simulink model "Signalmodulation"  (R2024b)
settings: Solver=VariableStepAuto  StartTime=0.0  StopTime=10.0  RelTol=1e-3
libraries: commchan3 x1, simulink x1, dspfdesign x1
settings Model: Creator=pc  LastModifiedBy=pc
settings DebuggingCC: UnconnectedInputMsg=warning  UnconnectedOutputMsg=warning  UnconnectedLineMsg=warning
settings ModelReferenceCC: EnableRefExpFcnMdlSchedulingChecks=on
settings RTWCC: GPUComputeCapability=3.5  DLArmComputeVersion=19.05

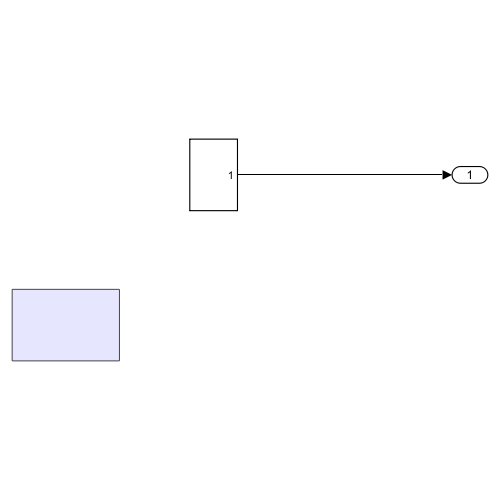
[thumbnail: Simulink's stored preview of the top-level diagram]
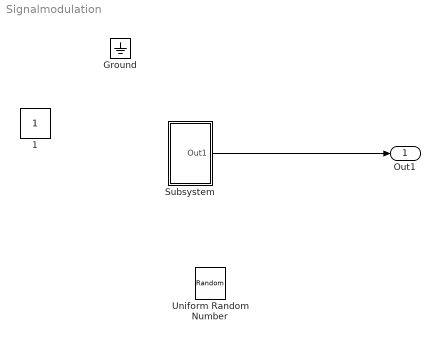
== system Signalmodulation ==
  Subsystem : Subsystem
  Out1 : Outport
  "1 " : Constant  IOType=siggen
  Ground : Ground  IOType=siggen
  Uniform Random Number : UniformRandomNumber  IOType=siggen  SampleTime=0
  wires:
  Subsystem/1(Out1) -> Out1/1

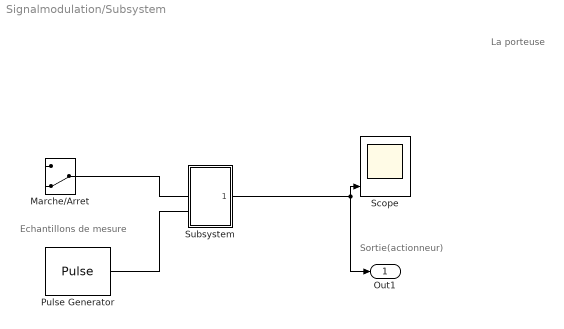
== system Signalmodulation/Subsystem ==
  note: La porteuse
  note: Sortie(actionneur)
  note: Echantillons de mesure
  Marche/Arret : ManualSwitch  CurrentSetting=0
  Pulse Generator : DiscretePulseGenerator  PulseType=Time based  PulseWidth=50
  Scope : Scope  NumInputPorts=3
  Subsystem : Subsystem
  Out1 : Outport
  wires:
  Subsystem/1(Received signal) -> Out1/1, Scope/3
  Marche/Arret/1 -> ?
  Pulse Generator/1 -> ?
  ? -> Scope/1
  ? -> Scope/2

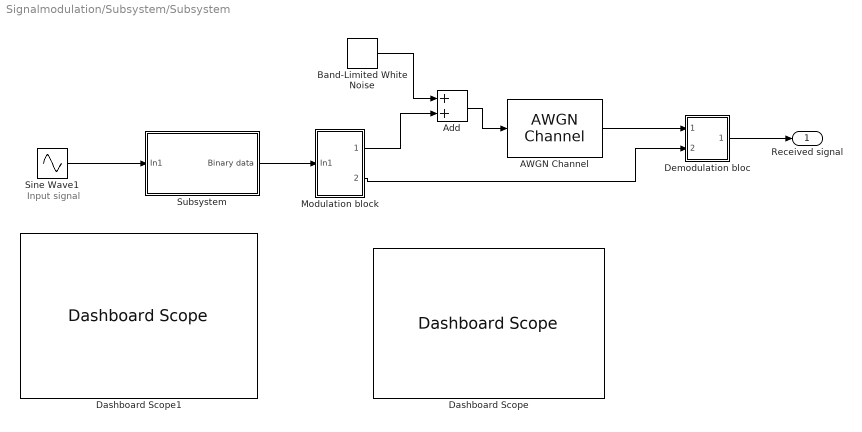
== system Signalmodulation/Subsystem/Subsystem ==
  note: Input signal
  AWGN Channel : commchan3/AWGN Channel  LegacyMode=on  NoiseMethod="Signal to noise ratio  (SNR)"  noiseMode="Signal to noise ratio  (SNR)"  EbNo=0  EsNo=10  SNR=10  BitsPerSymbol=1  SignalPower=1  SamplesPerSymbol=1  SymbolPeriod=1  VarianceSource=Parameter  Variance=1  RandomStream=Global stream  Seed=67  SimulateUsing=Code generation
  Add : Sum
  Band-Limited White Noise : simulink/Sources/Band-Limited White Noise  Cov=[0.1]  Ts=0.1  seed=[23341]
  Dashboard Scope : DashboardScope
  Dashboard Scope1 : DashboardScope
  Demodulation bloc : Subsystem
  Modulation block : Subsystem
  Sine Wave1 : Sin  SampleTime=0
  Subsystem : Subsystem
  Received signal : Outport
  wires:
  Subsystem/1("Binary data ") -> Modulation block/1(In1)
  Add/1 -> AWGN Channel/1
  Sine Wave1/1 -> Subsystem/1(In1)
  AWGN Channel/1 -> Demodulation bloc/1(In1)
  Modulation block/2(Out3) -> Demodulation bloc/2(In2)
  Demodulation bloc/1(Out1) -> Received signal/1
  Band-Limited White Noise/1 -> Add/1
  Modulation block/1(Out1) -> Add/2

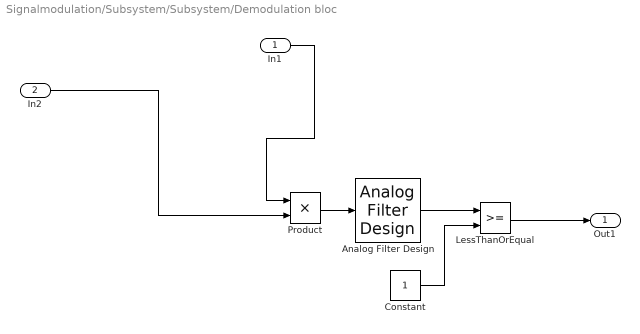
== system Signalmodulation/Subsystem/Subsystem/Demodulation bloc ==
  In1 : Inport
  In2 : Inport  Port=2
  Analog Filter Design : dspfdesign/Analog Filter Design  method=Chebyshev I  filttype=Lowpass  N=8  Wlo=10  Whi=80  Rp=2  Rs=40
  Constant : Constant
  LessThanOrEqual : RelationalOperator  OutDataTypeStr=boolean  RndMeth=Simplest  InputSameDT=off
  Product : Product
  Out1 : Outport
  wires:
  Product/1 -> Analog Filter Design/1
  Analog Filter Design/1 -> LessThanOrEqual/1
  In1/1 -> Product/1
  Constant/1 -> LessThanOrEqual/2
  LessThanOrEqual/1 -> Out1/1
  In2/1 -> Product/2

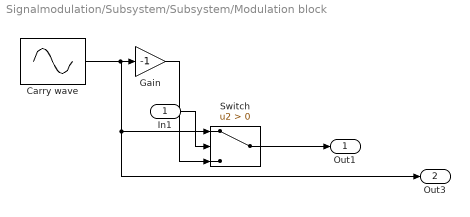
== system Signalmodulation/Subsystem/Subsystem/Modulation block ==
  In1 : Inport
  Carry wave : Sin  Amplitude=3  Frequency=8*pi  SampleTime=0.0001
  Gain : Gain  Gain=-1
  Switch : Switch  Criteria=u2 > Threshold  SaturateOnIntegerOverflow=off  InputSameDT=off
  Out1 : Outport
  Out3 : Outport  Port=2
  wires:
  Switch/1 -> Out1/1
  Gain/1 -> Switch/3
  Carry wave/1 -> Gain/1, Out3/1, Switch/1
  In1/1 -> Switch/2

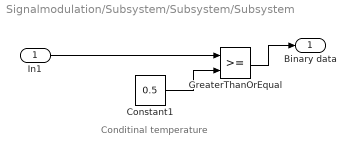
== system Signalmodulation/Subsystem/Subsystem/Subsystem ==
  note: Conditinal temperature
  In1 : Inport
  Constant1 : Constant  Value=0.5
  GreaterThanOrEqual : RelationalOperator  OutDataTypeStr=boolean  RndMeth=Simplest  InputSameDT=off
  "Binary data " : Outport
  wires:
  GreaterThanOrEqual/1 -> "Binary data "/1
  Constant1/1 -> GreaterThanOrEqual/2
  In1/1 -> GreaterThanOrEqual/1
